simulink model "Motor_control_DTC"  (R2017b)
settings: Solver=VariableStepAuto  StartTime=0.0  StopTime=10  RelTol=1e-3
values from neighbouring files (symbols this model uses):
  Kd = 3    [control_params.m]
  Ki = 7    [control_params.m]
  Kp = 10    [control_params.m]
  max_PID = 10    [control_params.m]
  min_PID = 0    [control_params.m]
  Mref_switch = 1    [control_params.m]
  PolePairs = 2    [control_params.m]
  Psierr = 0.02    [control_params.m]
  Psiref = 1    [control_params.m]
  Trqerr = 1    [control_params.m]
  Tsamp = 0.0001    [control_params.m]
libraries: misc_lib x5, controller_lib x4, electricdrivelib x1, autolibim x1, coordinate_transform_lib x1
settings Model: Creator=Máté  LastModifiedBy=Máté

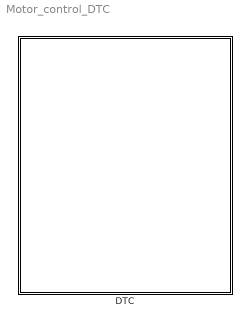
== system Motor_control_DTC ==
  DTC : Subsystem

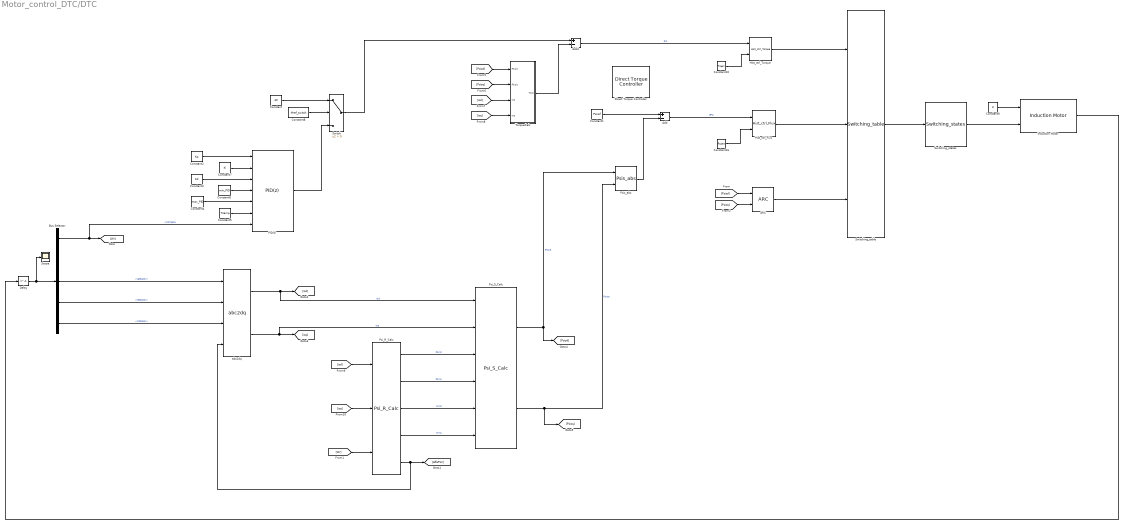
== system Motor_control_DTC/DTC ==
  ARC : controller_lib/ARC
  Add : Sum  Inputs=+-
  Add1 : Sum  Inputs=+-
  Bus Selector : BusSelector  OutputSignals=MtrSpd,MtrTrq,IaStator,IbStator,IcStator
  Constant : Constant  Value=40
  Constant1 : Constant  Value=Psiref
  Constant10 : Constant  Value=Trqerr
  Constant16 : Constant  Value=Psierr
  Constant2 : Constant  Value=Kp
  Constant3 : Constant  Value=Kd
  Constant4 : Constant  Value=max_PID
  Constant5 : Constant  Value=Tsamp
  Constant6 : Constant  Value=min_PID
  Constant7 : Constant  Value=Ki
  Constant8 : Constant  Value=Mref_switch
  Constant9 : Constant  Value=3  VectorParams1D=off
  Delay : Delay  DelayLength=1
  Direct Torque Controller : electricdrivelib/Fundamental Drive Blocks/Direct Torque Controller  OverrideUsingVariant=Detailed  modulationType=Hysteresis  T_bw=0.5  kp_Te=1.5  ki_Te=100  F_bw=0.01  kp_Flux=250  ki_Flux=4000  Ts_DTFC=20e-6  Ts=1e-6  freq_max=20000  car_freq=20000  fc_bus=50  Rss=0.435  in_flux=0.3  p=2
      settings: SourceProductName=Simscape Power Systems  SourceProductBaseCode=PS
  Hist_ctrl_Flux : controller_lib/Hist_ctrl_Flux
  Hist_ctrl_Torque : controller_lib/Hist_ctrl_Torque
  Induction Motor : autolibim/Induction Motor  port_config=Torque  Zs=[1.7 5.4e-3]  Zr="[1.41  4.9e-3]"  Lm=92.6e-3  P=2  theta_init=0  omega_init=0  mechanical=[0.001 0 0]
      settings: SourceProductName=Powertrain Blockset  SourceProductBaseCode=PW
  PID(z) : controller_lib/PID(z)
  Psi_R_Calc : misc_lib/Psi_R_Calc
  Psi_S_Calc : misc_lib/Psi_S_Calc
  Psis_abs : misc_lib/Psis_abs
  Scope : Scope
  Switch : Switch  Criteria=u2 > Threshold
  "Switching_states " : misc_lib/Switching_states 
  Switching_table : misc_lib/Switching_table
  TorqueCalc : Subsystem
  "abc2dq " : coordinate_transform_lib/abc2dq 
  wires:
  PID(z)/1 -> Switch/3
  Constant/1 -> Switch/1
  Constant1/1 -> Add/1
  Add/1 -> Hist_ctrl_Flux/1  "dPsi"
  ARC/1 -> Switching_table/3
  Add1/1 -> Hist_ctrl_Torque/1  "dm"
  Constant2/1 -> PID(z)/1
  Constant3/1 -> PID(z)/3
  Constant4/1 -> PID(z)/5
  Constant5/1 -> PID(z)/6
  Constant6/1 -> PID(z)/4
  Constant7/1 -> PID(z)/2
  Constant8/1 -> Switch/2
  Switch/1 -> Add1/1
  Bus Selector/3 -> "abc2dq "/1  "<IaStator>"
  Bus Selector/4 -> "abc2dq "/2  "<IbStator>"
  Bus Selector/5 -> "abc2dq "/3  "<IcStator>"
  Bus Selector/1 -> PID(z)/7, [Wr]  "<MtrSpd>"
  TorqueCalc/1(Tout) -> Add1/2
  Psi_R_Calc/5 -> "abc2dq "/4, [AlfaPsir]
  Psi_R_Calc/1 -> Psi_S_Calc/3  "Psird"
  Psi_R_Calc/2 -> Psi_S_Calc/4  "Psirq"
  Psi_R_Calc/3 -> Psi_S_Calc/5  "imrd"
  Psi_R_Calc/4 -> Psi_S_Calc/6  "imrq"
  [Wr] -> Psi_R_Calc/3
  Constant16/1 -> Hist_ctrl_Flux/2
  Switching_table/1 -> "Switching_states "/1
  "abc2dq "/1 -> Psi_S_Calc/1, [isd]  "isd"
  "abc2dq "/2 -> Psi_S_Calc/2, [isq]  "isq"
  Psi_S_Calc/1 -> Psis_abs/1, [Psisd]  "Psisd"
  Psi_S_Calc/2 -> Psis_abs/2, [Psisq]  "Psisq"
  [Psisd] -> TorqueCalc/1(Psisd)
  [Psisq] -> TorqueCalc/2(Psisq)
  [isq] -> TorqueCalc/4(isq)
  [isd] -> TorqueCalc/3(isd)
  [isd] -> Psi_R_Calc/1
  [isq] -> Psi_R_Calc/2
  [Psisd] -> ARC/1
  [Psisq] -> ARC/2
  Hist_ctrl_Torque/1 -> Switching_table/1
  Hist_ctrl_Flux/1 -> Switching_table/2
  Psis_abs/1 -> Add/2
  "Switching_states "/1 -> Induction Motor/2
  Constant9/1 -> Induction Motor/1
  Induction Motor/1 -> Delay/1
  Delay/1 -> Scope/1, Bus Selector/1
  Constant10/1 -> Hist_ctrl_Torque/2

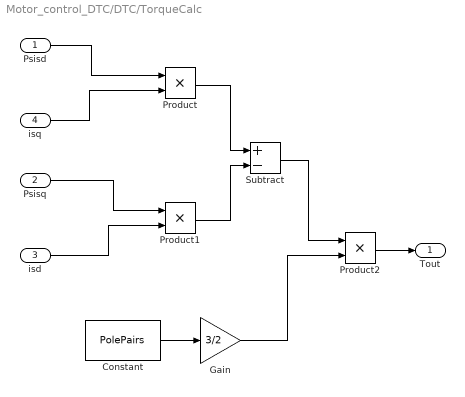
== system Motor_control_DTC/DTC/TorqueCalc ==
  Psisd : Inport
  Psisq : Inport  Port=2
  isd : Inport  Port=3
  isq : Inport  Port=4
  Constant : Constant  Value=PolePairs
  Gain : Gain  Gain=3/2
  Product : Product
  Product1 : Product
  Product2 : Product
  Subtract : Sum  Inputs=+-
  Tout : Outport
  wires:
  Constant/1 -> Gain/1
  Psisd/1 -> Product/1
  isq/1 -> Product/2
  Psisq/1 -> Product1/1
  isd/1 -> Product1/2
  Product/1 -> Subtract/1
  Product1/1 -> Subtract/2
  Subtract/1 -> Product2/1
  Gain/1 -> Product2/2
  Product2/1 -> Tout/1
